simulink model "gm_HDLRegToVariable_vs"  (R2024a)
settings: Solver=FixedStepDiscrete  StartTime=0.0  StopTime=stopTime  RelTol=1e-3
values from neighbouring files (symbols this model uses):
  fs = 1    [testHeaderFull.m]
undefined symbols (not defined in the file or in its folder): clk, clk_enable, reset_x
libraries: simulink x12, dspsrcs4 x5, HDL_ieee_8021513 x2, whdlutilities x1, vivadosimlib x1
settings Model: Creator=cotti  LastModifiedBy=cotti
settings SolverCC: AutoInsertRateTranBlk=on
settings OptimizationCC: BlockReduction=off  ConditionallyExecuteInputs=off  DefaultParameterBehavior=Inlined  InheritOutputTypeSmallerThanSingle=on
settings DebuggingCC: AlgebraicLoopMsg=error  ArtificialAlgebraicLoopMsg=error  InheritedTsInSrcMsg=none  SingleTaskRateTransMsg=error  UnconnectedInputMsg=warning  UnconnectedOutputMsg=warning  UnconnectedLineMsg=warning
settings HardwareCC: ProdBitPerPointer=32  ProdBitPerSizeT=32  ProdBitPerPtrDiffT=32  ProdLargestAtomicFloat=None  ProdIntDivRoundTo=Undefined  ProdEndianess=Unspecified  ProdWordSize=32  ProdHWDeviceType=ASIC/FPGA->ASIC/FPGA  TargetBitPerLong=64  TargetBitPerPointer=64  TargetBitPerSizeT=64  TargetBitPerPtrDiffT=64  TargetLongLongMode=on  TargetIntDivRoundTo=Zero  TargetEndianess=LittleEndian  TargetWordSize=64  TargetHWDeviceType=Custom Processor->MATLAB Host Computer  ProdEqTarget=off

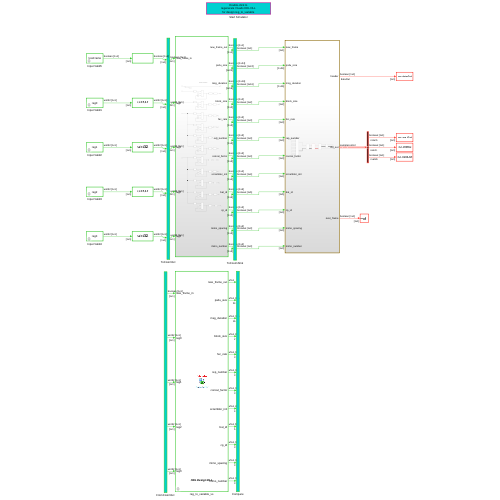
[thumbnail: Simulink's stored preview of the top-level diagram]
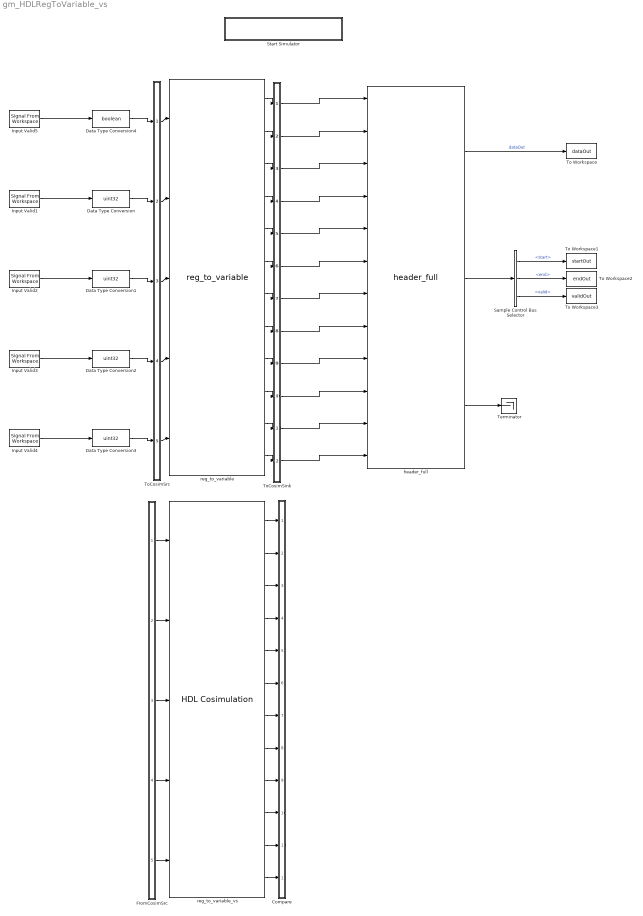
== system gm_HDLRegToVariable_vs ==
  Compare : Subsystem
      mask Display: disp('')
  Data Type Conversion{,1..3} (4 alike) : DataTypeConversion  OutDataTypeStr=uint32  SaturateOnIntegerOverflow=off  RndMeth=Floor
  Data Type Conversion4 : DataTypeConversion  OutDataTypeStr=boolean  SaturateOnIntegerOverflow=off  RndMeth=Floor
  FromCosimSrc : Subsystem
      mask Display: disp('')
  Input Valid1 : dspsrcs4/Signal From Workspace  X=reg0  Ts=1/fs  nsamps=1  OutputAfterFinalValue=Setting to zero  ignoreOrWarnInputAndFrameLengths=off  OutputFrames=off
  Input Valid2 : dspsrcs4/Signal From Workspace  X=reg1  Ts=1/fs  nsamps=1  OutputAfterFinalValue=Setting to zero  ignoreOrWarnInputAndFrameLengths=off  OutputFrames=off
  Input Valid3 : dspsrcs4/Signal From Workspace  X=reg2  Ts=1/fs  nsamps=1  OutputAfterFinalValue=Setting to zero  ignoreOrWarnInputAndFrameLengths=off  OutputFrames=off
  Input Valid4 : dspsrcs4/Signal From Workspace  X=reg3  Ts=1/fs  nsamps=1  OutputAfterFinalValue=Setting to zero  ignoreOrWarnInputAndFrameLengths=off  OutputFrames=off
  Input Valid5 : dspsrcs4/Signal From Workspace  X=newFrame  Ts=1/fs  nsamps=1  OutputAfterFinalValue=Setting to zero  ignoreOrWarnInputAndFrameLengths=off  OutputFrames=off
  Sample Control Bus Selector : whdlutilities/Sample Control Bus Selector  OutputSignals=start,end,valid
  Start Simulator : Subsystem
      settings: OpenFcn=|
      | cosimDirName = pwd;
      | cd 'hdl_prj/hdlsrc/HDLHeaderFull';
      | [s,r] = system('vivado -mode batch -source gm_HDLHeaderFull_vs.tcl','-echo');
      | cd (cosimDirName);
      | clear cosimDirName;
      | if s
      |    error('Failed to create Vivado HDL design DLL using script gm_HDLHeaderFull_vs.tcl.');
      | end
      mask Display: disp('Double-click to\nregenerate Vivado HDL DLL\nfor design reg_to_variable')
  Terminator : Terminator
  To Workspace : ToWorkspace  VariableName=dataOut  SampleTime=1/(8*fs)
      settings: Save2DSignal=2-D array (concatenate along first dimension)
  To Workspace1 : ToWorkspace  VariableName=startOut  SampleTime=1/(8*fs)
      settings: Save2DSignal=2-D array (concatenate along first dimension)
  To Workspace2 : ToWorkspace  VariableName=endOut  SampleTime=1/(8*fs)
      settings: Save2DSignal=2-D array (concatenate along first dimension)
  To Workspace3 : ToWorkspace  VariableName=validOut  SampleTime=1/(8*fs)
      settings: Save2DSignal=2-D array (concatenate along first dimension)
  ToCosimSink : Subsystem
      mask Display: disp('')
  ToCosimSrc : Subsystem
      mask Display: disp('')
  header_full : HDL_ieee_8021513/header_full  SystemSampleTime=-1  VariantActivationTime=update diagram  AllowFlexibleInterface=on  Latency=0  AutoFrameSizeCalculation=off
      settings: LibrarySourceBlock=|
      | hdlsllib/Ports &
      | Subsystems/Subsystem
  reg_to_variable : HDL_ieee_8021513/reg_to_variable  SystemSampleTime=-1  VariantActivationTime=update diagram  AllowFlexibleInterface=on  Latency=0  AutoFrameSizeCalculation=off
      settings: SourceProductName=HDL IEEE 8021513
  reg_to_variable_vs : vivadosimlib/HDL Cosimulation  PortPaths=/reg_to_variable/new_frame_in;/reg_to_variable/reg0;/reg_to_variable/reg1;/reg_to_variable/reg2;/reg_to_variable/reg3;/reg_to_variable/new_frame_out;/reg_to_variable/psdu_size;/reg_to_variable/msg_duration;/reg_to_variable/block_size;/reg_to_variable/fec_rate;/reg_to_variable/rep_number;/reg_to_variable/concat_factor;/reg_to_variable/scrambler_init;/reg_to_variable/bat_id;/reg_to_variable/cp_id;/reg_to_variable/mimo_spacing;/reg_to_variable/mimo_number  PortModes=[1 1 1 1 1 2 2 2 2 2 2 2 2 2 2 2 2 ]  PortTimes=[-1 -1 -1 -1 -1 1.0000000000000000209225608301284726753266340892878361046314239502e-08 1.0000000000000000209225608301284726753266340892878361046314239502e-08 1.0000000000000000209225608301284726753266340892878361046314239502e-08 1.0000000000000000209225608301284726753266340892878361046314239502e-08 1.0000000000000000209225608301284726753266340892878361046314239502e-08 1.0000000000000000209225608301284726753266340892878361046314239502e-08 1.0000000000000000209225608301284726753266340892878361046314239502e-08 1.0000000000000000209225608301284726753266340892878361046314239502e-08 1.0000000000000000209225608301284726753266340892878361046314239502e-08 1.0000000000000000209225608301284726753266340892878361046314239502e-08 1.0000000000000000209225608301284726753266340892878361046314239502e-08 1.0000000000000000209225608301284726753266340892878361046314239502e-08 ]  PortSigns=[-1 -1 -1 -1 -1 0 -1 -1 -1 -1 -1 -1 -1 -1 -1 -1 -1 ]  PortFracLengths=[0,0,0,0,0,0,0,0,0,0,0,0,0,0,0,0,0]  PortWordLengths=[-1,-1,-1,-1,-1,1,1,1,1,1,1,1,1,1,1,1,1]  PortHDLWordSizes=[1,32,32,32,32,1,1,1,1,1,1,1,1,1,1,1,1]  CommLocal=on  CommSharedMemory=on  CommPortNumber=4449  CommShowInfo=on  ClockPaths=clk;clk_enable;reset_x;  ClockModes=[2 4 3]  ClockTimes=[1e-08 3.7e-08 2.7e-08]  TclPostSimCommand="puts \"done\""  TimingMode=ns  TimingScaleFactor=1000000000  idxCellArray={'UNUSED_VAR'}  CosimBypass=Full Simulation  AllowDirectFeedthrough=on  ProductName=EDA Simulator Link VS  RunAutoTimescale=off  HdlClocks=0  PreRunTime=40  PreRunTimeUnit=ns
  wires:
  Sample Control Bus Selector/2 -> To Workspace2/1  "<end>"
  header_full/1 -> To Workspace/1  "dataOut"
  Sample Control Bus Selector/3 -> To Workspace3/1  "<valid>"
  Sample Control Bus Selector/1 -> To Workspace1/1  "<start>"
  header_full/2 -> Sample Control Bus Selector/1
  Input Valid4/1 -> Data Type Conversion3/1
  Input Valid3/1 -> Data Type Conversion2/1
  Input Valid2/1 -> Data Type Conversion1/1
  Input Valid1/1 -> Data Type Conversion/1
  Input Valid5/1 -> Data Type Conversion4/1
  header_full/3 -> Terminator/1
  ToCosimSrc/1(out1) -> reg_to_variable/1
  ToCosimSrc/2(out2) -> reg_to_variable/2
  ToCosimSrc/3(out3) -> reg_to_variable/3
  ToCosimSrc/4(out4) -> reg_to_variable/4
  ToCosimSrc/5(out5) -> reg_to_variable/5
  reg_to_variable/1 -> ToCosimSink/1(in1)
  reg_to_variable/2 -> ToCosimSink/2(in2)
  reg_to_variable/3 -> ToCosimSink/3(in3)
  reg_to_variable/4 -> ToCosimSink/4(in4)
  reg_to_variable/5 -> ToCosimSink/5(in5)
  reg_to_variable/6 -> ToCosimSink/6(in6)
  reg_to_variable/7 -> ToCosimSink/7(in7)
  reg_to_variable/8 -> ToCosimSink/8(in8)
  reg_to_variable/9 -> ToCosimSink/9(in9)
  reg_to_variable/10 -> ToCosimSink/10(in10)
  reg_to_variable/11 -> ToCosimSink/11(in11)
  reg_to_variable/12 -> ToCosimSink/12(in12)
  Data Type Conversion4/1 -> ToCosimSrc/1(in1)
  Data Type Conversion/1 -> ToCosimSrc/2(in2)
  Data Type Conversion1/1 -> ToCosimSrc/3(in3)
  Data Type Conversion2/1 -> ToCosimSrc/4(in4)
  Data Type Conversion3/1 -> ToCosimSrc/5(in5)
  ToCosimSink/1(out1) -> header_full/1
  ToCosimSink/2(out2) -> header_full/2
  ToCosimSink/3(out3) -> header_full/3
  ToCosimSink/4(out4) -> header_full/4
  ToCosimSink/5(out5) -> header_full/5
  ToCosimSink/6(out6) -> header_full/6
  ToCosimSink/7(out7) -> header_full/7
  ToCosimSink/8(out8) -> header_full/8
  ToCosimSink/9(out9) -> header_full/9
  ToCosimSink/10(out10) -> header_full/10
  ToCosimSink/11(out11) -> header_full/11
  ToCosimSink/12(out12) -> header_full/12
  FromCosimSrc/1(out1) -> reg_to_variable_vs/1
  FromCosimSrc/2(out2) -> reg_to_variable_vs/2
  FromCosimSrc/3(out3) -> reg_to_variable_vs/3
  FromCosimSrc/4(out4) -> reg_to_variable_vs/4
  FromCosimSrc/5(out5) -> reg_to_variable_vs/5
  reg_to_variable_vs/1 -> Compare/1(in1)
  reg_to_variable_vs/2 -> Compare/2(in2)
  reg_to_variable_vs/3 -> Compare/3(in3)
  reg_to_variable_vs/4 -> Compare/4(in4)
  reg_to_variable_vs/5 -> Compare/5(in5)
  reg_to_variable_vs/6 -> Compare/6(in6)
  reg_to_variable_vs/7 -> Compare/7(in7)
  reg_to_variable_vs/8 -> Compare/8(in8)
  reg_to_variable_vs/9 -> Compare/9(in9)
  reg_to_variable_vs/10 -> Compare/10(in10)
  reg_to_variable_vs/11 -> Compare/11(in11)
  reg_to_variable_vs/12 -> Compare/12(in12)

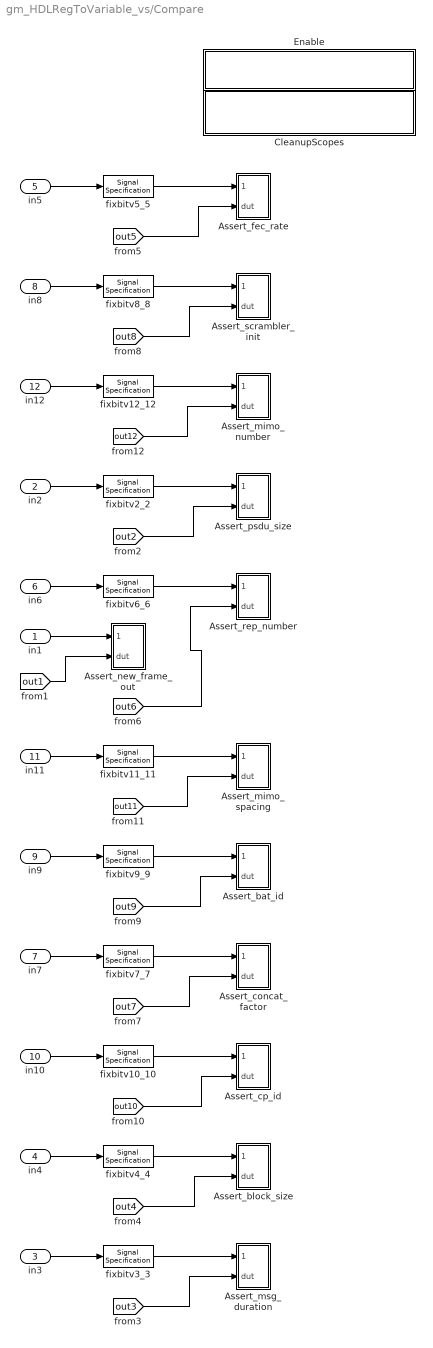
== system gm_HDLRegToVariable_vs/Compare ==
  in1 : Inport
  in2 : Inport  Port=2
  in3 : Inport  Port=3
  in4 : Inport  Port=4
  in5 : Inport  Port=5
  in6 : Inport  Port=6
  in7 : Inport  Port=7
  in8 : Inport  Port=8
  in9 : Inport  Port=9
  in10 : Inport  Port=10
  in11 : Inport  Port=11
  in12 : Inport  Port=12
  Assert_bat_id : Subsystem
      settings: LibrarySourceBlock=hdlmdlgenlib/AssertEq
  Assert_block_size : Subsystem
      settings: LibrarySourceBlock=hdlmdlgenlib/AssertEq
  Assert_concat_factor : Subsystem
      settings: LibrarySourceBlock=hdlmdlgenlib/AssertEq
  Assert_cp_id : Subsystem
      settings: LibrarySourceBlock=hdlmdlgenlib/AssertEq
  Assert_fec_rate : Subsystem
      settings: LibrarySourceBlock=hdlmdlgenlib/AssertEq
  Assert_mimo_number : Subsystem
      settings: LibrarySourceBlock=hdlmdlgenlib/AssertEq
  Assert_mimo_spacing : Subsystem
      settings: LibrarySourceBlock=hdlmdlgenlib/AssertEq
  Assert_msg_duration : Subsystem
      settings: LibrarySourceBlock=hdlmdlgenlib/AssertEq
  Assert_new_frame_out : Subsystem
      settings: LibrarySourceBlock=hdlmdlgenlib/AssertEq
  Assert_psdu_size : Subsystem
      settings: LibrarySourceBlock=hdlmdlgenlib/AssertEq
  Assert_rep_number : Subsystem
      settings: LibrarySourceBlock=hdlmdlgenlib/AssertEq
  Assert_scrambler_init : Subsystem
      settings: LibrarySourceBlock=hdlmdlgenlib/AssertEq
  CleanupScopes : Subsystem
      settings: OpenFcn=|
      | blkName = gcb; %self block
      | idx = regexp(blkName, '/CleanupScopes$', 'once');
      | blkParent = blkName(1:idx-1);
      | blks=find_system(blkParent, 'LookUnderMasks', 'all','blocktype', 'Scope');
      | for itr = 1:length(blks)
      | 	 hScopeCfg = get_param(blks{itr},'ScopeConfiguration');
      | 	 hScopeCfg.Visible = ~ hScopeCfg.Visible;
      | end
      | drawnow;
      mask Display: fprintf(message('hdlcoder:cosim:vnl_dblclick').getString());
  Enable : Subsystem
      settings: OpenFcn=|
      | blkName = gcb;
      | idx = regexp(blkName, '/Enable$', 'once');
      | blkParent = blkName(1:idx-1);
      | blks=find_system(blkParent, 'LookUnderMasks', 'all','blocktype', 'Assertion');
      | e = get_param(blks{1}, 'Enabled');
      | if strcmp(e, 'on'), f= 'off';, else, f = 'on';, end
      | for ii=1:length(blks), set_param(blks{ii}, 'Enabled', f);, end
      | set_param(gcb, 'MaskDisplay',['fprintf(message(''hdlcoder:cosim:vnl_dblclick_assertions'',','''',upper(e),'''',').getString())']);
      mask Display: fprintf(message('hdlcoder:cosim:vnl_dblclick_assertions','OFF').getString());
  fixbitv10_10 : SignalSpecification  OutDataTypeStr=fixdt(0,1,0)  Dimensions=3
  fixbitv11_11 : SignalSpecification  OutDataTypeStr=fixdt(0,1,0)  Dimensions=3
  fixbitv12_12 : SignalSpecification  OutDataTypeStr=fixdt(0,1,0)  Dimensions=3
  fixbitv2_2 : SignalSpecification  OutDataTypeStr=fixdt(0,1,0)  Dimensions=24
  fixbitv3_3 : SignalSpecification  OutDataTypeStr=fixdt(0,1,0)  Dimensions=16
  fixbitv4_4 : SignalSpecification  OutDataTypeStr=fixdt(0,1,0)  Dimensions=2
  fixbitv5_5 : SignalSpecification  OutDataTypeStr=fixdt(0,1,0)  Dimensions=3
  fixbitv6_6 : SignalSpecification  OutDataTypeStr=fixdt(0,1,0)  Dimensions=3
  fixbitv7_7 : SignalSpecification  OutDataTypeStr=fixdt(0,1,0)  Dimensions=3
  fixbitv8_8 : SignalSpecification  OutDataTypeStr=fixdt(0,1,0)  Dimensions=4
  fixbitv9_9 : SignalSpecification  OutDataTypeStr=fixdt(0,1,0)  Dimensions=5
  wires:
  [out3] -> Assert_msg_duration/2(dut)
  fixbitv3_3/1 -> Assert_msg_duration/1(cosim)
  fixbitv4_4/1 -> Assert_block_size/1(cosim)
  fixbitv10_10/1 -> Assert_cp_id/1(cosim)
  [out2] -> Assert_psdu_size/2(dut)
  fixbitv9_9/1 -> Assert_bat_id/1(cosim)
  in9/1 -> fixbitv9_9/1
  fixbitv6_6/1 -> Assert_rep_number/1(cosim)
  fixbitv5_5/1 -> Assert_fec_rate/1(cosim)
  [out12] -> Assert_mimo_number/2(dut)
  [out1] -> Assert_new_frame_out/2(dut)
  [out7] -> Assert_concat_factor/2(dut)
  in6/1 -> fixbitv6_6/1
  [out10] -> Assert_cp_id/2(dut)
  in7/1 -> fixbitv7_7/1
  in12/1 -> fixbitv12_12/1
  [out4] -> Assert_block_size/2(dut)
  in11/1 -> fixbitv11_11/1
  in2/1 -> fixbitv2_2/1
  [out5] -> Assert_fec_rate/2(dut)
  in10/1 -> fixbitv10_10/1
  in8/1 -> fixbitv8_8/1
  fixbitv2_2/1 -> Assert_psdu_size/1(cosim)
  [out6] -> Assert_rep_number/2(dut)
  in4/1 -> fixbitv4_4/1
  in3/1 -> fixbitv3_3/1
  fixbitv12_12/1 -> Assert_mimo_number/1(cosim)
  [out9] -> Assert_bat_id/2(dut)
  in5/1 -> fixbitv5_5/1
  in1/1 -> Assert_new_frame_out/1(cosim)
  fixbitv8_8/1 -> Assert_scrambler_init/1(cosim)
  [out8] -> Assert_scrambler_init/2(dut)
  fixbitv11_11/1 -> Assert_mimo_spacing/1(cosim)
  [out11] -> Assert_mimo_spacing/2(dut)
  fixbitv7_7/1 -> Assert_concat_factor/1(cosim)

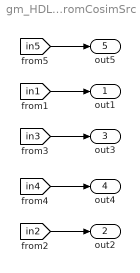
== system gm_HDLRegToVariable_vs/FromCosimSrc ==
  out1 : Outport
  out2 : Outport  Port=2
  out3 : Outport  Port=3
  out4 : Outport  Port=4
  out5 : Outport  Port=5
  wires:
  [in2] -> out2/1
  [in4] -> out4/1
  [in3] -> out3/1
  [in1] -> out1/1
  [in5] -> out5/1

== system gm_HDLRegToVariable_vs/Start Simulator ==

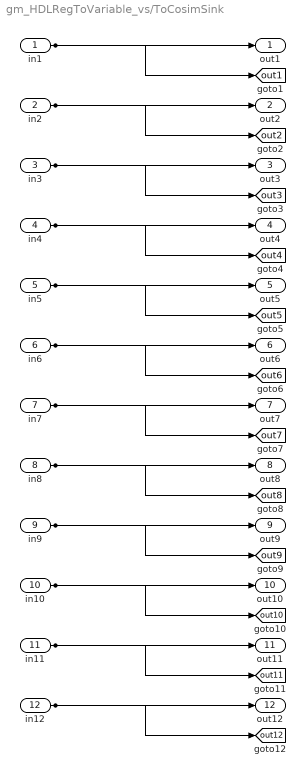
== system gm_HDLRegToVariable_vs/ToCosimSink ==
  in1 : Inport
  in2 : Inport  Port=2
  in3 : Inport  Port=3
  in4 : Inport  Port=4
  in5 : Inport  Port=5
  in6 : Inport  Port=6
  in7 : Inport  Port=7
  in8 : Inport  Port=8
  in9 : Inport  Port=9
  in10 : Inport  Port=10
  in11 : Inport  Port=11
  in12 : Inport  Port=12
  out1 : Outport
  out2 : Outport  Port=2
  out3 : Outport  Port=3
  out4 : Outport  Port=4
  out5 : Outport  Port=5
  out6 : Outport  Port=6
  out7 : Outport  Port=7
  out8 : Outport  Port=8
  out9 : Outport  Port=9
  out10 : Outport  Port=10
  out11 : Outport  Port=11
  out12 : Outport  Port=12
  tag scope: out10=global, out11=global, out12=global, out1=global, out2=global, out3=global, out4=global, out5=global, out6=global, out7=global, out8=global, out9=global
  wires:
  in1/1 -> out1/1, [out1]
  in2/1 -> out2/1, [out2]
  in3/1 -> out3/1, [out3]
  in4/1 -> out4/1, [out4]
  in5/1 -> out5/1, [out5]
  in6/1 -> out6/1, [out6]
  in7/1 -> out7/1, [out7]
  in8/1 -> out8/1, [out8]
  in9/1 -> out9/1, [out9]
  in10/1 -> out10/1, [out10]
  in11/1 -> out11/1, [out11]
  in12/1 -> out12/1, [out12]

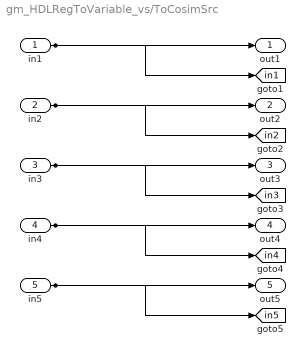
== system gm_HDLRegToVariable_vs/ToCosimSrc ==
  in1 : Inport
  in2 : Inport  Port=2
  in3 : Inport  Port=3
  in4 : Inport  Port=4
  in5 : Inport  Port=5
  out1 : Outport
  out2 : Outport  Port=2
  out3 : Outport  Port=3
  out4 : Outport  Port=4
  out5 : Outport  Port=5
  tag scope: in1=global, in2=global, in3=global, in4=global, in5=global
  wires:
  in1/1 -> out1/1, [in1]
  in2/1 -> out2/1, [in2]
  in3/1 -> out3/1, [in3]
  in4/1 -> out4/1, [in4]
  in5/1 -> out5/1, [in5]

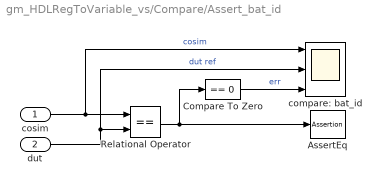
== system gm_HDLRegToVariable_vs/Compare/Assert_bat_id ==
  cosim : Inport
  dut : Inport  Port=2
  AssertEq : Assertion
  Compare To Zero : simulink/Logic and Bit Operations/Compare To Zero  relop===  OutDataTypeStr=boolean
  Relational Operator : RelationalOperator  Operator===  OutDataTypeStr=boolean  InputSameDT=off
  compare: bat_id : Scope  NumInputPorts=3
  wires:
  Compare To Zero/1 -> compare: bat_id/3  "err"
  Relational Operator/1 -> Compare To Zero/1, AssertEq/1
  cosim/1 -> compare: bat_id/1, Relational Operator/1  "cosim"
  dut/1 -> compare: bat_id/2, Relational Operator/2  "dut ref"

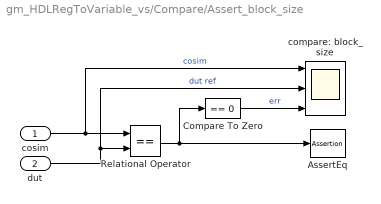
== system gm_HDLRegToVariable_vs/Compare/Assert_block_size ==
  cosim : Inport
  dut : Inport  Port=2
  AssertEq : Assertion
  Compare To Zero : simulink/Logic and Bit Operations/Compare To Zero  relop===  OutDataTypeStr=boolean
  Relational Operator : RelationalOperator  Operator===  OutDataTypeStr=boolean  InputSameDT=off
  compare: block_size : Scope  NumInputPorts=3
  wires:
  Compare To Zero/1 -> compare: block_size/3  "err"
  Relational Operator/1 -> Compare To Zero/1, AssertEq/1
  cosim/1 -> compare: block_size/1, Relational Operator/1  "cosim"
  dut/1 -> compare: block_size/2, Relational Operator/2  "dut ref"

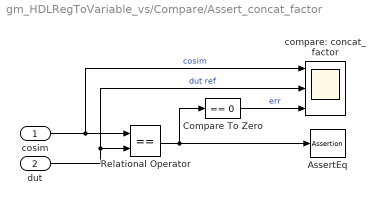
== system gm_HDLRegToVariable_vs/Compare/Assert_concat_factor ==
  cosim : Inport
  dut : Inport  Port=2
  AssertEq : Assertion
  Compare To Zero : simulink/Logic and Bit Operations/Compare To Zero  relop===  OutDataTypeStr=boolean
  Relational Operator : RelationalOperator  Operator===  OutDataTypeStr=boolean  InputSameDT=off
  compare: concat_factor : Scope  NumInputPorts=3
  wires:
  Compare To Zero/1 -> compare: concat_factor/3  "err"
  Relational Operator/1 -> Compare To Zero/1, AssertEq/1
  cosim/1 -> compare: concat_factor/1, Relational Operator/1  "cosim"
  dut/1 -> compare: concat_factor/2, Relational Operator/2  "dut ref"

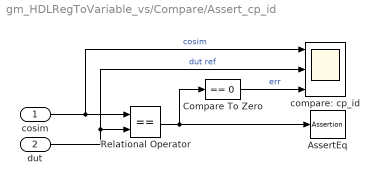
== system gm_HDLRegToVariable_vs/Compare/Assert_cp_id ==
  cosim : Inport
  dut : Inport  Port=2
  AssertEq : Assertion
  Compare To Zero : simulink/Logic and Bit Operations/Compare To Zero  relop===  OutDataTypeStr=boolean
  Relational Operator : RelationalOperator  Operator===  OutDataTypeStr=boolean  InputSameDT=off
  compare: cp_id : Scope  NumInputPorts=3
  wires:
  Compare To Zero/1 -> compare: cp_id/3  "err"
  Relational Operator/1 -> Compare To Zero/1, AssertEq/1
  cosim/1 -> compare: cp_id/1, Relational Operator/1  "cosim"
  dut/1 -> compare: cp_id/2, Relational Operator/2  "dut ref"

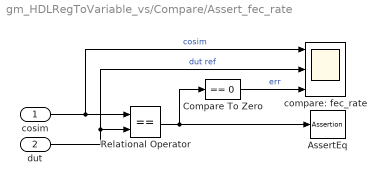
== system gm_HDLRegToVariable_vs/Compare/Assert_fec_rate ==
  cosim : Inport
  dut : Inport  Port=2
  AssertEq : Assertion
  Compare To Zero : simulink/Logic and Bit Operations/Compare To Zero  relop===  OutDataTypeStr=boolean
  Relational Operator : RelationalOperator  Operator===  OutDataTypeStr=boolean  InputSameDT=off
  compare: fec_rate : Scope  NumInputPorts=3
  wires:
  Compare To Zero/1 -> compare: fec_rate/3  "err"
  Relational Operator/1 -> Compare To Zero/1, AssertEq/1
  cosim/1 -> compare: fec_rate/1, Relational Operator/1  "cosim"
  dut/1 -> compare: fec_rate/2, Relational Operator/2  "dut ref"

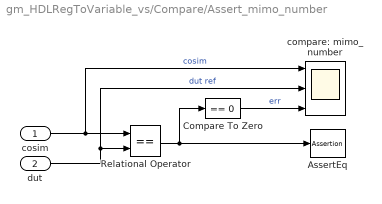
== system gm_HDLRegToVariable_vs/Compare/Assert_mimo_number ==
  cosim : Inport
  dut : Inport  Port=2
  AssertEq : Assertion
  Compare To Zero : simulink/Logic and Bit Operations/Compare To Zero  relop===  OutDataTypeStr=boolean
  Relational Operator : RelationalOperator  Operator===  OutDataTypeStr=boolean  InputSameDT=off
  compare: mimo_number : Scope  NumInputPorts=3
  wires:
  Compare To Zero/1 -> compare: mimo_number/3  "err"
  Relational Operator/1 -> Compare To Zero/1, AssertEq/1
  cosim/1 -> compare: mimo_number/1, Relational Operator/1  "cosim"
  dut/1 -> compare: mimo_number/2, Relational Operator/2  "dut ref"

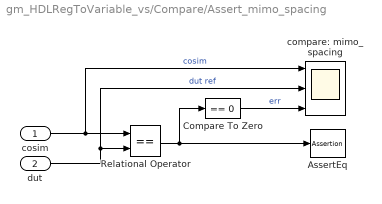
== system gm_HDLRegToVariable_vs/Compare/Assert_mimo_spacing ==
  cosim : Inport
  dut : Inport  Port=2
  AssertEq : Assertion
  Compare To Zero : simulink/Logic and Bit Operations/Compare To Zero  relop===  OutDataTypeStr=boolean
  Relational Operator : RelationalOperator  Operator===  OutDataTypeStr=boolean  InputSameDT=off
  compare: mimo_spacing : Scope  NumInputPorts=3
  wires:
  Compare To Zero/1 -> compare: mimo_spacing/3  "err"
  Relational Operator/1 -> Compare To Zero/1, AssertEq/1
  cosim/1 -> compare: mimo_spacing/1, Relational Operator/1  "cosim"
  dut/1 -> compare: mimo_spacing/2, Relational Operator/2  "dut ref"

== system gm_HDLRegToVariable_vs/Compare/Assert_msg_duration ==
  cosim : Inport
  dut : Inport  Port=2
  AssertEq : Assertion
  Compare To Zero : simulink/Logic and Bit Operations/Compare To Zero  relop===  OutDataTypeStr=boolean
  Relational Operator : RelationalOperator  Operator===  OutDataTypeStr=boolean  InputSameDT=off
  compare: msg_duration : Scope  NumInputPorts=3
  wires:
  Compare To Zero/1 -> compare: msg_duration/3  "err"
  Relational Operator/1 -> Compare To Zero/1, AssertEq/1
  cosim/1 -> compare: msg_duration/1, Relational Operator/1  "cosim"
  dut/1 -> compare: msg_duration/2, Relational Operator/2  "dut ref"

== system gm_HDLRegToVariable_vs/Compare/Assert_new_frame_out ==
  cosim : Inport
  dut : Inport  Port=2
  AssertEq : Assertion
  Compare To Zero : simulink/Logic and Bit Operations/Compare To Zero  relop===  OutDataTypeStr=boolean
  Relational Operator : RelationalOperator  Operator===  OutDataTypeStr=boolean  InputSameDT=off
  compare: new_frame_out : Scope  NumInputPorts=3
  wires:
  Compare To Zero/1 -> compare: new_frame_out/3  "err"
  Relational Operator/1 -> Compare To Zero/1, AssertEq/1
  cosim/1 -> compare: new_frame_out/1, Relational Operator/1  "cosim"
  dut/1 -> compare: new_frame_out/2, Relational Operator/2  "dut ref"

== system gm_HDLRegToVariable_vs/Compare/Assert_psdu_size ==
  cosim : Inport
  dut : Inport  Port=2
  AssertEq : Assertion
  Compare To Zero : simulink/Logic and Bit Operations/Compare To Zero  relop===  OutDataTypeStr=boolean
  Relational Operator : RelationalOperator  Operator===  OutDataTypeStr=boolean  InputSameDT=off
  compare: psdu_size : Scope  NumInputPorts=3
  wires:
  Compare To Zero/1 -> compare: psdu_size/3  "err"
  Relational Operator/1 -> Compare To Zero/1, AssertEq/1
  cosim/1 -> compare: psdu_size/1, Relational Operator/1  "cosim"
  dut/1 -> compare: psdu_size/2, Relational Operator/2  "dut ref"

== system gm_HDLRegToVariable_vs/Compare/Assert_rep_number ==
  cosim : Inport
  dut : Inport  Port=2
  AssertEq : Assertion
  Compare To Zero : simulink/Logic and Bit Operations/Compare To Zero  relop===  OutDataTypeStr=boolean
  Relational Operator : RelationalOperator  Operator===  OutDataTypeStr=boolean  InputSameDT=off
  compare: rep_number : Scope  NumInputPorts=3
  wires:
  Compare To Zero/1 -> compare: rep_number/3  "err"
  Relational Operator/1 -> Compare To Zero/1, AssertEq/1
  cosim/1 -> compare: rep_number/1, Relational Operator/1  "cosim"
  dut/1 -> compare: rep_number/2, Relational Operator/2  "dut ref"

== system gm_HDLRegToVariable_vs/Compare/Assert_scrambler_init ==
  cosim : Inport
  dut : Inport  Port=2
  AssertEq : Assertion
  Compare To Zero : simulink/Logic and Bit Operations/Compare To Zero  relop===  OutDataTypeStr=boolean
  Relational Operator : RelationalOperator  Operator===  OutDataTypeStr=boolean  InputSameDT=off
  compare: scrambler_init : Scope  NumInputPorts=3
  wires:
  Compare To Zero/1 -> compare: scrambler_init/3  "err"
  Relational Operator/1 -> Compare To Zero/1, AssertEq/1
  cosim/1 -> compare: scrambler_init/1, Relational Operator/1  "cosim"
  dut/1 -> compare: scrambler_init/2, Relational Operator/2  "dut ref"

== system gm_HDLRegToVariable_vs/Compare/CleanupScopes ==

== system gm_HDLRegToVariable_vs/Compare/Enable ==
